simulink model "InvClarkTran"  (R2022b)
settings: Solver=FixedStepDiscrete  StartTime=0.0  StopTime=10.0  FixedStep=0.000001  RelTol=1e-3
settings Model: Creator=yll  LastModifiedBy=yll

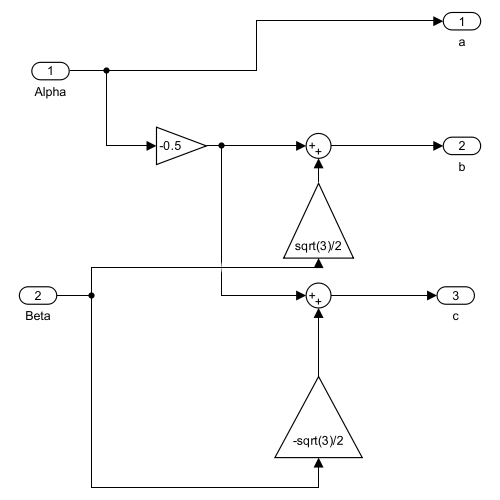
[thumbnail: Simulink's stored preview of the top-level diagram]
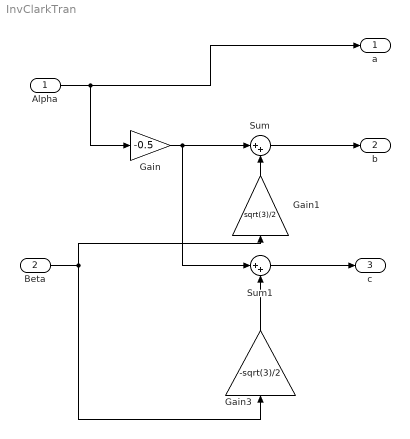
== system InvClarkTran ==
  Alpha : Inport
  Beta : Inport  Port=2
  Gain : Gain  Gain=-0.5
  Gain1 : Gain  Gain=sqrt(3)/2
  Gain3 : Gain  Gain=-sqrt(3)/2
  Sum : Sum  Inputs=|++
  Sum1 : Sum  Inputs=|++
  a : Outport
  b : Outport  Port=2
  c : Outport  Port=3
  wires:
  Alpha/1 -> a/1, Gain/1
  Gain1/1 -> Sum/2
  Gain/1 -> Sum1/1, Sum/1
  Gain3/1 -> Sum1/2
  Beta/1 -> Gain1/1, Gain3/1
  Sum/1 -> b/1
  Sum1/1 -> c/1
